simulink model "robulink"  (R2013a)
settings: Solver=ode3  SolverMode=SingleTasking  StartTime=0.0  StopTime=inf  RelTol=1e-3
undefined symbols (not defined in the file or in its folder): Normalized
libraries: legonxtlib x10
settings Model: SimulationMode=external  ExtModeTrigDuration=2  Creator=leeclement  LastModifiedBy=leeclement
settings OptimizationCC: OptimizeModelRefInitCode=on  LifeSpan=1
settings DebuggingCC: SolverPrmCheckMsg=none  StrictBusMsg=Warning
settings HardwareCC: ProdLargestAtomicInteger=Long  ProdLargestAtomicFloat=Float  ProdEndianess=LittleEndian  ProdHWDeviceType=ARM Compatible->ARM 7
settings RTWCC: SystemTargetFile=realtime.tlc  GenerateMakefile=off  TemplateMakefile=realtime.tmf  Description=Run on Target Hardware  RTWVerbose=off  ProcessScript=realtime_make_rtw_hook
settings STFCustomTargetCC: TargetLibSuffix=.a  GenerateSampleERTMain=on  ERTCustomFileBanners=on  SupportNonInlinedSFcns=off  SupportVariableSizeSignals=on  MATLABClassNameForMDSCustomization=Simulink.SoftwareTarget.ERTCustomization  SystemTargetFile=realtime.tlc
settings ERTTargetCC: ParMdlRefBuildCompliant=off  CompOptLevelCompliant=off  ConcurrentExecutionCompliant=off  CombineOutputUpdateFcns=off  ERTFirstTimeCompliant=off  SupportContinuousTime=on  SupportVariableSizeSignals=on  ModelStepFunctionPrototypeControlCompliant=off  CPPClassGenCompliant=off  ExtMode=on  ExtModeTransport=2  ExtModeMexFile=ext_serial_win32_comm_no_acks_rtt  ExtModeMexArgs=0 7 9600  ERTSrcFileBannerTemplate=realtime_code_template.cgt  ERTHdrFileBannerTemplate=realtime_code_template.cgt  ERTDataSrcFileTemplate=realtime_code_template.cgt  ERTDataHdrFileTemplate=realtime_code_template.cgt  ERTCustomFileTemplate=realtime_file_process.tlc

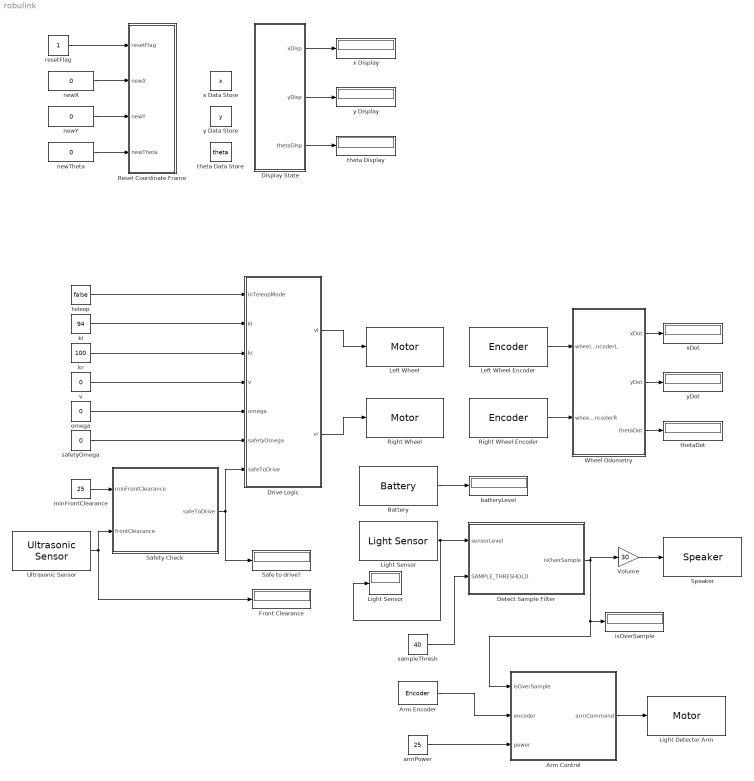
== system robulink ==
  Arm Control : MATLAB Function  TreatAsAtomicUnit=on
  Arm Encoder : legonxtlib/Encoder  portNumber=B  opMode=Reset at each sample time  sampleTime=0.1
  Battery : legonxtlib/Battery  sampleTime=0.1
  Detect Sample Filter : MATLAB Function  TreatAsAtomicUnit=on
  Display State : MATLAB Function  TreatAsAtomicUnit=on
  Drive Logic : MATLAB Function  TreatAsAtomicUnit=on
  Front Clearance : Display
  Left Wheel : legonxtlib/Motor  sportNumber=C  sstopAction=Brake
  Left Wheel Encoder : legonxtlib/Encoder  portNumber=C  opMode=Reset at each sample time  sampleTime=0.1
  Light Detector Arm : legonxtlib/Motor  sportNumber=B  sstopAction=Brake
  Light Sensor : legonxtlib/Light Sensor  portNumber=2  outputMode=Normalized (0 -100)  lightOn=on  sampleTime=0.1
  "Light Sensor " : Display
  Reset Coordinate Frame : MATLAB Function  TreatAsAtomicUnit=on
  "Right Wheel " : legonxtlib/Motor  sportNumber=A  sstopAction=Brake
  "Right Wheel Encoder " : legonxtlib/Encoder  portNumber=A  opMode=Reset at each sample time  sampleTime=0.1
  Safe to drive? : Display
  Safety Check : MATLAB Function  TreatAsAtomicUnit=on
  Speaker : legonxtlib/Speaker  sinputMode=Volume only  sspeakerFreq=1000  sspeakerVolume=50  sspeakerDuration=500
  Ultrasonic Sensor : legonxtlib/Ultrasonic Sensor  PortNumber=1  sampleTime=0.1
  Volume : Gain  Gain=30
  Wheel Odometry : MATLAB Function  TreatAsAtomicUnit=on
  armPower : Constant  Value=25
  batteryLevel : Display
  isOverSample : Display
  kl : Constant  Value=94
  kr : Constant  Value=100
  minFrontClearance : Constant  Value=25
  newTheta : Constant  Value=0
  newX : Constant  Value=0
  newY : Constant  Value=0
  omega : Constant  Value=0
  resetFlag : Constant
  safetyOmega : Constant  Value=0
  sampleThresh : Constant  Value=40
  teleop : Constant  Value=false
  theta Data Store : DataStoreMemory  DataStoreName=theta  ReadBeforeWriteMsg=warning  WriteAfterWriteMsg=warning  WriteAfterReadMsg=warning  OutDataTypeStr=double
  theta Display : Display
  thetaDot : Display
  v : Constant  Value=0
  x Data Store : DataStoreMemory  DataStoreName=x  ReadBeforeWriteMsg=warning  WriteAfterWriteMsg=warning  WriteAfterReadMsg=warning  OutDataTypeStr=double
  x Display : Display
  xDot : Display
  y Data Store : DataStoreMemory  DataStoreName=y  ReadBeforeWriteMsg=warning  WriteAfterWriteMsg=warning  WriteAfterReadMsg=warning  OutDataTypeStr=double
  y Display : Display
  yDot : Display
  wires:
  Drive Logic/1(vl) -> Left Wheel/1
  Drive Logic/2(vr) -> "Right Wheel "/1
  Ultrasonic Sensor/1 -> Front Clearance/1, Safety Check/2(frontClearance)
  "Right Wheel Encoder "/1 -> Wheel Odometry/2(wheelEncoderR)
  Left Wheel Encoder/1 -> Wheel Odometry/1(wheelEncoderL)
  Display State/3(thetaDisp) -> theta Display/1
  Display State/1(xDisp) -> x Display/1
  Display State/2(yDisp) -> y Display/1
  resetFlag/1 -> Reset Coordinate Frame/1(resetFlag)
  kl/1 -> Drive Logic/2(kl)
  kr/1 -> Drive Logic/3(kr)
  newX/1 -> Reset Coordinate Frame/2(newX)
  newY/1 -> Reset Coordinate Frame/3(newY)
  newTheta/1 -> Reset Coordinate Frame/4(newTheta)
  v/1 -> Drive Logic/4(v)
  omega/1 -> Drive Logic/5(omega)
  teleop/1 -> Drive Logic/1(inTeleopMode)
  Safety Check/1(safeToDrive) -> Safe to drive?/1, Drive Logic/7(safeToDrive)
  minFrontClearance/1 -> Safety Check/1(minFrontClearance)
  safetyOmega/1 -> Drive Logic/6(safetyOmega)
  Light Sensor/1 -> "Light Sensor "/1, Detect Sample Filter/1(sensorLevel)
  Detect Sample Filter/1(isOverSample) -> Volume/1, Arm Control/1(isOverSample), isOverSample/1
  Volume/1 -> Speaker/1
  Battery/1 -> batteryLevel/1
  Wheel Odometry/1(xDot) -> xDot/1
  Wheel Odometry/2(yDot) -> yDot/1
  Wheel Odometry/3(thetaDot) -> thetaDot/1
  sampleThresh/1 -> Detect Sample Filter/2(SAMPLE_THRESHOLD)
  Arm Encoder/1 -> Arm Control/2(encoder)
  armPower/1 -> Arm Control/3(power)
  Arm Control/1(armCommand) -> Light Detector Arm/1

== matlab function robulink/Wheel Odometry ==
  data: wheelEncoderL input; wheelEncoderR input; x data_store_memory; y data_store_memory; theta data_store_memory; xDot output; yDot output; thetaDot output
function [xDot, yDot, thetaDot] = wheelOdometry(wheelEncoderL, wheelEncoderR)
% PURPOSE:  Computes new state update based on wheel encoder values and
%           previous state
%
% INPUTS:   wheelEncoderL   -   encoder value of left wheel  (degrees)
%           wheelEncoderR   -   encoder value of right wheel (degrees)
%           x, y, theta     -   previous state (global variables)
%
% OUTPUTS:  Linear and rotational velocities
%
% NOTE: Assumes wheel encoders are reset at every time step
    
     global x;
     global y;
     global theta;

    % Constants
    sampleTime = 0.1;           % seconds
    
    wheelRadius = 0.04;         % meters
    wheelSeparation = 0.15;     % meters
    
    % Kinematics
    % Negative sign because motors installed upside down
    omegaL = -double(wheelEncoderL) / sampleTime;
    omegaR = -double(wheelEncoderR) / sampleTime;
    
    B = [ 0.5 * wheelRadius * cosd(theta),  0.5 * wheelRadius * cosd(theta);
          0.5 * wheelRadius * sind(theta),  0.5 * wheelRadius * sind(theta);
          wheelRadius / wheelSeparation,    - wheelRadius / wheelSeparation];
      
    update = sampleTime * B * (pi/180) * [omegaR; omegaL];
    
    rates = B * (pi/180) * [omegaR; omegaL];
    xDot = rates(1);
    yDot = rates(2);
    thetaDot = rates(3);
    
    
    % /60 because of weird unit issue?
    x = x + update(1);
    y = y + update(2);
    theta = theta + update(3) * 180/pi;
    
    if theta > 180
        theta = theta - 360;
    elseif theta <= -180
        theta = theta + 360;
    end
end

== matlab function robulink/Drive Logic ==
  data: inTeleopMode input; kl input; kr input; vl output; vr output; v input; omega input; safetyOmega input; theta data_store_memory; safeToDrive input
function [vl, vr] = driveLogic(inTeleopMode, kl, kr, v, omega, safetyOmega, safeToDrive)
    d = 0.15;       % distance between left-right wheels
%     kl = 94.25;     % gain to relate wheel speed [m/s] to applied command [dimensionless]
%     kr = 100;
    
    % for safety, start by assigning wheel speeds to zero
    vl = 0;
    vr = 0;
    
    if ~safeToDrive && ~inTeleopMode
        v = 0;
        omega = safetyOmega;
    end
    
    vl =  -kl*(v - 0.5*d*omega);  % left wheel command
    vr =  -kr*(v + 0.5*d*omega);  % right wheel commmand
    
%     vl = 0;
%     vr = 0;
end

== matlab function robulink/Display State ==
  data: xDisp output; yDisp output; thetaDisp output; x data_store_memory; y data_store_memory; theta data_store_memory
function [xDisp,yDisp,thetaDisp] = displayState
    global x;
    global y;
    global theta;
    
    xDisp = x;
    yDisp = y;
    thetaDisp = theta;
end

== matlab function robulink/Safety Check ==
  data: minFrontClearance input; frontClearance input; safeToDrive output
function safeToDrive = isSafeToDrive(minFrontClearance, frontClearance)    
    % Clearances are in cm
    
    safeToDrive = frontClearance >= minFrontClearance;
end

== matlab function robulink/Detect Sample Filter ==
  data: sensorLevel input; isOverSample output; SAMPLE_THRESHOLD input
function isOverSample = detectSample(sensorLevel, SAMPLE_THRESHOLD) %# codegen
%Rolling average filter
FILTER_SIZE = 10;
% %Light sensor threshold
% SAMPLE_THRESHOLD = 35;

persistent i buf bufSum;
if isempty(buf)
    buf = zeros(1,FILTER_SIZE);
    bufSum = 0;
    i = 1;
end
bufSum = bufSum - buf(i);
buf(i) = double(sensorLevel);
bufSum = bufSum + double(sensorLevel);
i = i + 1;
if i > numel(buf)
    i = 1;
end
avg = bufSum / numel(buf);

isOverSample = avg < SAMPLE_THRESHOLD;

== matlab function robulink/Reset Coordinate Frame ==
  data: resetFlag input; x data_store_memory; y data_store_memory; theta data_store_memory; newX input; newY input; newTheta input
function resetCoordFrame(resetFlag, newX, newY, newTheta)
    global x;
    global y;
    global theta;

    if(resetFlag == 1)
        x = newX;
        y = newY;
        theta = newTheta;
    end

end

== matlab function robulink/Arm Control ==
  data: isOverSample input; encoder input; armCommand output; power input
function armCommand = controlArm(isOverSample, encoder, power)
    % NB: Encoder is set to reset at every time step
    persistent prevDir;
    
    if isempty(prevDir)
        armDir = 1;
        prevDir = 1;
    else
        if(isOverSample)
            armDir = 0;
        else
            if encoder == 0
                armDir = -prevDir;
            else
                armDir = prevDir;
            end

            prevDir = armDir;
        end
    end
    
    armCommand = armDir * power;
end
